simulink library "TOWER_MASTER"  (Simulink 8.8)
settings: Solver=ode45  StartTime=0.0  StopTime=10.0  RelTol=1e-3  EnableMultiTasking=on
undefined symbols (not defined in the file): AC, AC2THRESHOLD, BF_WD_MASTER, GAS_WD_MASTER, GASAC, SIXOSEM_F_WD_AC_MASTER
libraries: cdsEpicsOut x163, cdsFilt x111, cdsTP x68, cdsFiltCtrl x56, cdsEpicsIn x47, cdsMuxMatrix x14, cdsRms x14, TOWER_MASTER x11, STATE_BIO_MASTER x8, cdsEpicsBinIn x6, cdsFunctionCall x4, VIS_LIB x2
(part 1 of 19)
settings Model: SuppressorTable=22 serialization::archive 11 0 3 0 0 0 11 0  Creator=controls  LastModifiedBy=controls

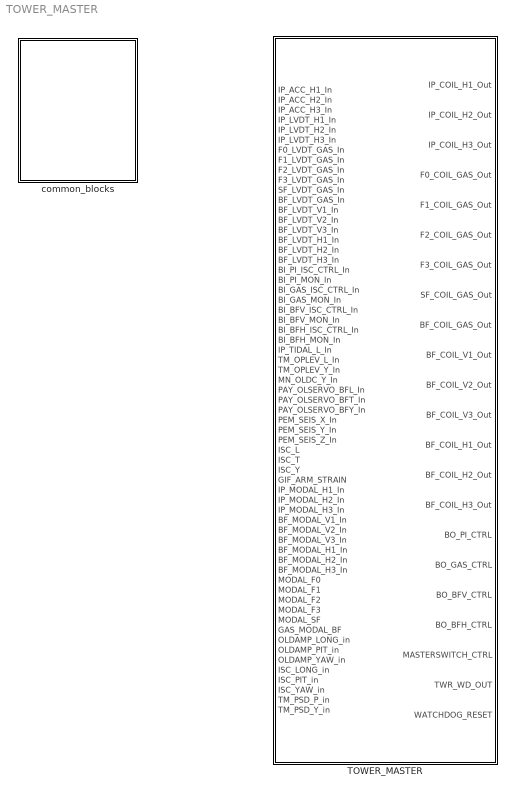
== system TOWER_MASTER ==
  TOWER_MASTER : Subsystem
  common_blocks : Subsystem

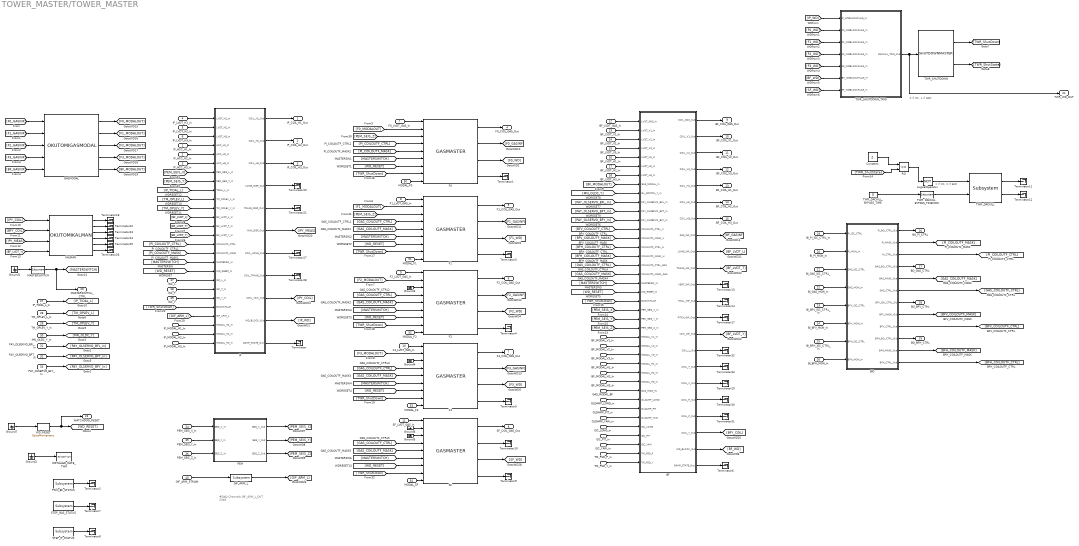
== system TOWER_MASTER/TOWER_MASTER ==
  note: 1 if OK, 0 if BAD
  note: 0 if OK, 1 if BAD
  note: #DAQ Channels
      | GIF_ARM_L_OUT 2048
  IP_ACC_H1_In : Inport
  IP_ACC_H2_In : Inport  Port=2
  IP_ACC_H3_In : Inport  Port=3
  IP_LVDT_H1_In : Inport  Port=4
  IP_LVDT_H2_In : Inport  Port=5
  IP_LVDT_H3_In : Inport  Port=6
  F0_LVDT_GAS_In : Inport  Port=7
  F1_LVDT_GAS_In : Inport  Port=8
  F2_LVDT_GAS_In : Inport  Port=9
  F3_LVDT_GAS_In : Inport  Port=10
  SF_LVDT_GAS_In : Inport  Port=11
  BF_LVDT_GAS_In : Inport  Port=12
  BF_LVDT_V1_In : Inport  Port=13
  BF_LVDT_V2_In : Inport  Port=14
  BF_LVDT_V3_In : Inport  Port=15
  BF_LVDT_H1_In : Inport  Port=16
  BF_LVDT_H2_In : Inport  Port=17
  BF_LVDT_H3_In : Inport  Port=18
  BI_PI_ISC_CTRL_In : Inport  Port=19
  BI_PI_MON_In : Inport  Port=20
  BI_GAS_ISC_CTRL_In : Inport  Port=21
  BI_GAS_MON_In : Inport  Port=22
  BI_BFV_ISC_CTRL_In : Inport  Port=23
  BI_BFV_MON_In : Inport  Port=24
  BI_BFH_ISC_CTRL_In : Inport  Port=25
  BI_BFH_MON_In : Inport  Port=26
  IP_TIDAL_L_In : Inport  Port=27
  TM_OPLEV_L_In : Inport  Port=28
  TM_OPLEV_Y_In : Inport  Port=29
  MN_OLDC_Y_In : Inport  Port=30
  PAY_OLSERVO_BFL_In : Inport  Port=31
  PAY_OLSERVO_BFT_In : Inport  Port=32
  PAY_OLSERVO_BFY_In : Inport  Port=33
  PEM_SEIS_X_In : Inport  Port=34
  PEM_SEIS_Y_In : Inport  Port=35
  PEM_SEIS_Z_In : Inport  Port=36
  ISC_L : Inport  Port=37
  ISC_T : Inport  Port=38
  ISC_Y : Inport  Port=39
  GIF_ARM_STRAIN : Inport  Port=40
  IP_MODAL_H1_In : Inport  Port=41
  IP_MODAL_H2_In : Inport  Port=42
  IP_MODAL_H3_In : Inport  Port=43
  BF_MODAL_V1_In : Inport  Port=44
  BF_MODAL_V2_In : Inport  Port=45
  BF_MODAL_V3_In : Inport  Port=46
  BF_MODAL_H1_In : Inport  Port=47
  BF_MODAL_H2_In : Inport  Port=48
  BF_MODAL_H3_In : Inport  Port=49
  MODAL_F0 : Inport  Port=50
  MODAL_F1 : Inport  Port=51
  MODAL_F2 : Inport  Port=52
  MODAL_F3 : Inport  Port=53
  MODAL_SF : Inport  Port=54
  GAS_MODAL_BF : Inport  Port=55
  OLDAMP_LONG_in : Inport  Port=56
  OLDAMP_PIT_in : Inport  Port=57
  OLDAMP_YAW_in : Inport  Port=58
  ISC_LONG_in : Inport  Port=59
  ISC_PIT_in : Inport  Port=60
  ISC_YAW_in : Inport  Port=61
  TM_PSD_P_in : Inport  Port=62
  TM_PSD_Y_in : Inport  Port=63
  BF : Subsystem
  BIO : Subsystem
  Constant : Constant  Value=2
  F{0..3} (4 alike) : TOWER_MASTER/common_blocks/GASMASTER
  GASMODAL : TOWER_MASTER/common_blocks/OKUTOMIGASMODAL
  GIF_ARM_L : cdsFilt/Subsystem  Tag=cdsFilt  Description=|
      | Purpose:                                                                                                                                                                                                                                  
      | Standard CDS IIR filter module.                                                                                                                                                                                                           
      |                                                                                                                                                                                                                                           
      | Operation:                                                                                                                                                                                                                                
      | Consists of 10 second order section IIR filters, plus a ramped gain stage. In FE code, also provides pre-defined test points and excitation channel inputs. The filter coefficients are defined in the LIGO system using the 'foton' tool.
      |                                                                                                                                                                                                                                           
      | Usage:                                                                                                                                                                                                                                    
      | Name the part with the desired filter module name.
      settings: AttributesFormatString=%<Tag>
  Ground{1..7} (7 alike) : Ground
  INSTALLED_DATE_TWR : cdsEpicsStringIn/EpicsStringIn  Tag=cdsEpicsStringIn  Description=cdsEpicsStringIn
      settings: AttributesFormatString=%<Tag>
  IP : Subsystem
  KALMAN : TOWER_MASTER/common_blocks/OKUTOMIKALMAN
  LogicalOperator : Logic  Operator=NOT  AllPortsSameDT=off  OutDataTypeStr=boolean
  MASTERSWITCH : cdsEpicsBinIn/Subsystem  Tag=cdsEpicsBinIn  Description=|
      | Purpose:                                                                            
      | Create an EPICS binary (0 or 1) input channel to the FE realtime controls.          
      |                                                                                     
      | Operation:                                                                          
      | Outputs value from an EPICS ai record. Value is binary input (bi Epics record type).
      |                                                                                     
      | Usage:                                                                              
      | Name the part with the desired EPICS channel name.
      settings: AttributesFormatString=%<Tag>
  PEM : Subsystem
  PICO_BF_STATUS : cdsEpicsIn/Subsystem  Tag=cdsEpicsIn  Description=|
      | Purpose:                                                                              
      | Create an EPICS input channel connection to the FE realtime controls.                 
      |                                                                                       
      | Operation:                                                                            
      | Outputs value from an EPICS ai record. Value is floating point with a precision of 3..
      |                                                                                       
      | Usage:                                                                                
      | Name the part with the desired EPICS channel name.
      settings: AttributesFormatString=%<Tag>
  RO : RelationalOperator  Operator===  OutDataTypeStr=boolean  RndMeth=Nearest
  SF : TOWER_MASTER/common_blocks/GASMASTER
  STEP_GAS_STATUS : cdsEpicsIn/Subsystem  Tag=cdsEpicsIn  Description=|
      | Purpose:                                                                              
      | Create an EPICS input channel connection to the FE realtime controls.                 
      |                                                                                       
      | Operation:                                                                            
      | Outputs value from an EPICS ai record. Value is floating point with a precision of 3..
      |                                                                                       
      | Usage:                                                                                
      | Name the part with the desired EPICS channel name.
      settings: AttributesFormatString=%<Tag>
  STEP_IP_STATUS : cdsEpicsIn/Subsystem  Tag=cdsEpicsIn  Description=|
      | Purpose:                                                                              
      | Create an EPICS input channel connection to the FE realtime controls.                 
      |                                                                                       
      | Operation:                                                                            
      | Outputs value from an EPICS ai record. Value is floating point with a precision of 3..
      |                                                                                       
      | Usage:                                                                                
      | Name the part with the desired EPICS channel name.
      settings: AttributesFormatString=%<Tag>
  TWR_DACKILL : cdsDacKill/Subsystem  Description=cdsDacKill
      settings: AttributesFormatString=%<Description>
  TWR_DACKILL_BYPASS_TIME : Constant  Value=0
  TWR_DACKILL_BYPASS_TIMEMON : cdsEpicsOut/Subsystem  Tag=cdsEpicsOutput  Description=|
      | Purpose:                                          
      | Output a FE signal to an EPICS channel.           
      |                                                   
      | Operation:                                        
      | Takes input value and passes it to EPICS record.  
      |                                                   
      | Usage:                                            
      | Name the part with the desired EPICS rrecord name.
      settings: AttributesFormatString=%<Tag>
  TWR_SHUTDOWN : TOWER_MASTER/common_blocks/SHUTDOWNMASTER
  TWR_SHUTDOWN_TRIG : Subsystem
  Terminator{,1..14,17..18,20..33} (31 alike) : Terminator
  WD_RESET : cdsEpicsMomentary/EpicsMomentary  Tag=cdsEpicsMomentary
      settings: AttributesFormatString=%<Tag>
  IP_COIL_H1_Out : Outport
  IP_COIL_H2_Out : Outport  Port=2
  IP_COIL_H3_Out : Outport  Port=3
  F0_COIL_GAS_Out : Outport  Port=4
  F1_COIL_GAS_Out : Outport  Port=5
  F2_COIL_GAS_Out : Outport  Port=6
  F3_COIL_GAS_Out : Outport  Port=7
  SF_COIL_GAS_Out : Outport  Port=8
  BF_COIL_GAS_Out : Outport  Port=9
  BF_COIL_V1_Out : Outport  Port=10
  BF_COIL_V2_Out : Outport  Port=11
  BF_COIL_V3_Out : Outport  Port=12
  BF_COIL_H1_Out : Outport  Port=13
  BF_COIL_H2_Out : Outport  Port=14
  BF_COIL_H3_Out : Outport  Port=15
  BO_PI_CTRL : Outport  Port=16
  BO_GAS_CTRL : Outport  Port=17
  BO_BFV_CTRL : Outport  Port=18
  BO_BFH_CTRL : Outport  Port=19
  MASTERSWITCH_CTRL : Outport  Port=20
  TWR_WD_OUT : Outport  Port=21
  WATCHDOG_RESET : Outport  Port=22
  wires:
  ISC_Y/1 -> IP/21(ISC_Y_in)
  ISC_T/1 -> IP/20(ISC_T_in)
  ISC_L/1 -> IP/19(ISC_L_in)
  GAS_MODAL_BF/1 -> BF/31(GAS_MOD_IN)
  BF_MODAL_H3_In/1 -> BF/30(MODAL_H3_In)
  BF_MODAL_H2_In/1 -> BF/29(MODAL_H2_In)
  BF_MODAL_H1_In/1 -> BF/28(MODAL_H1_In)
  BF_MODAL_V3_In/1 -> BF/27(MODAL_V3_In)
  BF_MODAL_V2_In/1 -> BF/26(MODAL_V2_In)
  BF_MODAL_V1_In/1 -> BF/25(MODAL_V1_In)
  [PEM_SEIS_Z] -> BF/24(PEM_SEIS_Z_In)
  [PEM_SEIS_Y] -> BF/23(PEM_SEIS_Y_In)
  [PEM_SEIS_X] -> BF/22(PEM_SEIS_X_In)
  [TWR_ShutDown] -> BF/21(BLOCKFLAG)
  [WD_RESET] -> BF/20(WD_RESET_In)
  [MASTERSWITCH] -> BF/19(MASTERSW_In)
  [GAS_COILOUTF_MASK] -> BF/18(COILOUTF_MASK_GAS)
  [GAS_COILOUTF_CTRL] -> BF/17(COILOUTF_CTRL_GAS)
  [BFH_COILOUTF_MASK] -> BF/16(COILOUTF_MASK_H)
  [BFH_COILOUTF_CTRL] -> BF/15(COILOUTF_CTRL_H)
  [BFV_COILOUTF_MASK] -> BF/14(COILOUTF_MASK_V)
  [BFV_COILOUTF_CTRL] -> BF/13(COILOUTF_CTRL_V)
  [PAY_OLSERVO_BFY_In] -> BF/12(PAY_OLSERVO_BFY_In)
  [PAY_OLSERVO_BFT_In] -> BF/11(PAY_OLSERVO_BFT_In)
  [PAY_OLSERVO_BFL_In] -> BF/10(PAY_OLSERVO_BFL_In)
  [MN_OLDC_Y] -> BF/9(OL_DCCTRL_Y_In)
  [BF_MODALOUT] -> BF/8(GAS_MODAL_In)
  BF_LVDT_H3_In/1 -> BF/7(LVDT_H3_In)
  BF_LVDT_H2_In/1 -> BF/6(LVDT_H2_In)
  BF_LVDT_H1_In/1 -> BF/5(LVDT_H1_In)
  BF_LVDT_V3_In/1 -> BF/4(LVDT_V3_In)
  BF_LVDT_V2_In/1 -> BF/3(LVDT_V2_In)
  BF_LVDT_V1_In/1 -> BF/2(LVDT_V1_In)
  BF_LVDT_GAS_In/1 -> BF/1(LVDT_GAS_In)
  TM_PSD_Y_in/1 -> BF/39(TM_PSD_Y)
  TM_PSD_P_in/1 -> BF/38(TM_PSD_P)
  ISC_PIT_in/1 -> BF/36(ISC_PIT)
  OLDAMP_YAW_in/1 -> BF/34(OLDAMP_YAW)
  OLDAMP_PIT_in/1 -> BF/33(OLDAMP_PIT)
  OLDAMP_LONG_in/1 -> BF/32(OLDAMP_LONG)
  ISC_YAW_in/1 -> BF/37(ISC_YAW)
  ISC_LONG_in/1 -> BF/35(ISC_LONG)
  [TWR_ShutDown] -> IP/22(BLOCKFLAG)
  [GIF_ARM_L] -> IP/23(GIF_ARM_L)
  MODAL_F3/1 -> F3/9
  MODAL_F2/1 -> F2/9
  MODAL_F1/1 -> F1/9
  MODAL_F0/1 -> F0/9
  IP_MODAL_H1_In/1 -> IP/24(MODAL_H1_In)
  IP_MODAL_H2_In/1 -> IP/25(MODAL_H2_In)
  IP_MODAL_H3_In/1 -> IP/26(MODAL_H3_In)
  RO/1 -> LogicalOperator/1
  [TWR_ShutState] -> RO/2
  Constant/1 -> RO/1
  TWR_SHUTDOWN/2 -> [TWR_ShutState]
  TWR_SHUTDOWN/1 -> [TWR_ShutDown]
  TWR_SHUTDOWN_TRIG/1(DACKILL_TRIG_Out) -> TWR_SHUTDOWN/1, TWR_WD_OUT/1
  TWR_DACKILL/2 -> Terminator12/1
  TWR_DACKILL/1 -> Terminator11/1
  TWR_DACKILL_BYPASS_TIME/1 -> TWR_DACKILL_BYPASS_TIMEMON/1
  TWR_DACKILL_BYPASS_TIMEMON/1 -> TWR_DACKILL/2
  LogicalOperator/1 -> TWR_DACKILL/1
  WD_RESET/1 -> [WD_RESET], WATCHDOG_RESET/1
  Ground7/1 -> WD_RESET/1
  MN_OLDC_Y_In/1 -> [MN_OLDC_Y]
  [IPY_MEAS] -> KALMAN/3
  [BF_LVDT_Y] -> KALMAN/4
  BF/20(COIL_Y_Out) -> [BFY_COIL]
  BF/17(COIL_V_Out) -> Terminator29/1
  BF/19(COIL_P_Out) -> Terminator31/1
  BF/18(COIL_R_Out) -> Terminator30/1
  BF/16(COIL_T_Out) -> Terminator33/1
  BF/15(COIL_L_Out) -> Terminator32/1
  BF/21(WD_BLOCK_Out) -> [BF_WD]
  BF/14(YAW_INF_Out) -> [BF_LVDT_Y]
  IP/11(DAMP_STATE_Out) -> Terminator/1
  IP/10(WD_BLOCK_Out) -> [IP_WD]
  IP/5(TRANS_DISP_Out) -> Terminator21/1
  IP/4(LONG_DISP_Out) -> Terminator20/1
  IP/9(COIL_YAW_Out) -> [IPY_COIL]
  IP/8(COIL_TRANS_Out) -> Terminator28/1
  IP/7(COIL_LONG_Out) -> Terminator27/1
  IP/6(YAW_DISP_Out) -> [IPY_MEAS]
  IP/3(COIL_H3_Out) -> IP_COIL_H3_Out/1
  KALMAN/6 -> Terminator26/1
  KALMAN/5 -> Terminator25/1
  KALMAN/4 -> Terminator24/1
  KALMAN/3 -> Terminator23/1
  KALMAN/2 -> Terminator22/1
  KALMAN/1 -> Terminator18/1
  [BFY_COIL] -> KALMAN/2
  [IPY_COIL] -> KALMAN/1
  BF/13(PITCH_INF_Out) -> Terminator17/1
  BF/12(ROLL_INF_Out) -> Terminator14/1
  BF/11(VERT_INF_Out) -> Terminator13/1
  BF/10(TRANS_INF_Out) -> [BF_LVDT_T]
  BF/9(LONG_INF_Out) -> [BF_LVDT_L]
  BF/8(GAS_INF_Out) -> [BF_GASINF]
  BF/7(COIL_H3_Out) -> BF_COIL_H3_Out/1
  BF/6(COIL_H2_Out) -> BF_COIL_H2_Out/1
  BF/5(COIL_H1_Out) -> BF_COIL_H1_Out/1
  BF/4(COIL_V3_Out) -> BF_COIL_V3_Out/1
  BF/3(COIL_V2_Out) -> BF_COIL_V2_Out/1
  BF/2(COIL_V1_Out) -> BF_COIL_V1_Out/1
  BF/1(COIL_GAS_Out) -> BF_COIL_GAS_Out/1
  [F3_MODALOUT] -> F3/2
  [F2_MODALOUT] -> F2/2
  [F1_MODALOUT] -> F1/2
  [F0_MODALOUT] -> F0/2
  GASMODAL/4 -> [F3_MODALOUT]
  GASMODAL/2 -> [F1_MODALOUT]
  GASMODAL/3 -> [F2_MODALOUT]
  GASMODAL/5 -> [BF_MODALOUT]
  GASMODAL/1 -> [F0_MODALOUT]
  [BF_GASINF] -> GASMODAL/5
  [F0_GASINF] -> GASMODAL/1
  [F1_GASINF] -> GASMODAL/2
  [F3_GASINF] -> GASMODAL/4
  [F2_GASINF] -> GASMODAL/3
  F3/2 -> [F3_GASINF]
  F2/2 -> [F2_GASINF]
  F1/2 -> [F1_GASINF]
  F0/2 -> [F0_GASINF]
  F3_LVDT_GAS_In/1 -> F3/1
  F2_LVDT_GAS_In/1 -> F2/1
  F1_LVDT_GAS_In/1 -> F1/1
  F0_LVDT_GAS_In/1 -> F0/1
  F0/3 -> [F0_WD]
  F0/4 -> Terminator1/1
  F0/1 -> F0_COIL_GAS_Out/1
  BI_BFH_MON_In/1 -> BIO/8(BFH_MON_In)
  BI_BFH_ISC_CTRL_In/1 -> BIO/7(BFH_ISC_CTRL)
  BIO/10(BFH_BO_CTRL_Out) -> BO_BFH_CTRL/1
  BIO/12(BFH_CTRL_Out) -> [BFH_COILOUTF_CTRL]
  BIO/11(BFH_MASK_Out) -> [BFH_COILOUTF_MASK]
  BIO/9(BFV_CTRL_Out) -> [BFV_COILOUTF_CTRL]
  BIO/6(GAS_CTRL_Out) -> [GAS_COILOUTF_CTRL]
  BIO/3(PI_CTRL_Out) -> [PI_COILOUTF_CTRL]
  BIO/8(BFV_MASK_Out) -> [BFV_COILOUTF_MASK]
  BIO/5(GAS_MASK_Out) -> [GAS_COILOUTF_MASK]
  BIO/2(PI_MASK_Out) -> [PI_COILOUTF_MASK]
  BIO/7(BFV_BO_CTRL_Out) -> BO_BFV_CTRL/1
  BIO/4(GAS_BO_CTRL_Out) -> BO_GAS_CTRL/1
  BIO/1(PI_BO_CTRL_Out) -> BO_PI_CTRL/1
  BI_PI_MON_In/1 -> BIO/2(PI_MON_In)
  BI_PI_ISC_CTRL_In/1 -> BIO/1(PI_ISC_CTRL)
  BI_GAS_MON_In/1 -> BIO/4(GAS_MON_In)
  BI_BFV_MON_In/1 -> BIO/6(BFV_MON_In)
  BI_GAS_ISC_CTRL_In/1 -> BIO/3(GAS_ISC_CTRL)
  BI_BFV_ISC_CTRL_In/1 -> BIO/5(BFV_ISC_CTRL)
  [BF_WD] -> TWR_SHUTDOWN_TRIG/6(BF_WDBLOCKFLAG_In)
  [F3_WD] -> TWR_SHUTDOWN_TRIG/5(F3_WDBLOCKFLAG_In)
  [F2_WD] -> TWR_SHUTDOWN_TRIG/4(F2_WDBLOCKFLAG_In)
  [F1_WD] -> TWR_SHUTDOWN_TRIG/3(F1_WDBLOCKFLAG_In)
  [F0_WD] -> TWR_SHUTDOWN_TRIG/2(F0_WDBLOCKFLAG_In)
  [IP_WD] -> TWR_SHUTDOWN_TRIG/1(IP_WDBLOCKFLAG_In)
  F3/4 -> Terminator5/1
  F2/4 -> Terminator4/1
  F1/4 -> Terminator3/1
  F3/1 -> F3_COIL_GAS_Out/1
  F2/1 -> F2_COIL_GAS_Out/1
  F1/1 -> F1_COIL_GAS_Out/1
  F3/3 -> [F3_WD]
  F2/3 -> [F2_WD]
  F1/3 -> [F1_WD]
  MASTERSWITCH/1 -> MASTERSWITCH_CTRL/1, [MASTERSWITCH]
  IP/2(COIL_H2_Out) -> IP_COIL_H2_Out/1
  IP/1(COIL_H1_Out) -> IP_COIL_H1_Out/1
  IP_ACC_H3_In/1 -> IP/6(ACC_H3_In)
  IP_LVDT_H3_In/1 -> IP/3(LVDT_H3_In)
  IP_ACC_H1_In/1 -> IP/4(ACC_H1_In)
  IP_LVDT_H1_In/1 -> IP/1(LVDT_H1_In)
  IP_ACC_H2_In/1 -> IP/5(ACC_H2_In)
  IP_LVDT_H2_In/1 -> IP/2(LVDT_H2_In)
  PAY_OLSERVO_BFY_In/1 -> [PAY_OLSERVO_BFY_In]
  BF/22(DAMP_STATE_Out) -> Terminator6/1
  PEM/1(SEIS_X_Out) -> [PEM_SEIS_X]
  [PEM_SEIS_X] -> IP/7(PEM_SEIS_L_In)
  PEM/2(SEIS_Y_Out) -> [PEM_SEIS_Y]
  PEM/3(SEIS_Z_Out) -> [PEM_SEIS_Z]
  [PEM_SEIS_Y] -> IP/8(PEM_SEIS_T_In)
  PAY_OLSERVO_BFL_In/1 -> [PAY_OLSERVO_BFL_In]
  PAY_OLSERVO_BFT_In/1 -> [PAY_OLSERVO_BFT_In]
  PEM_SEIS_Y_In/1 -> PEM/2(SEIS_Y_In)
  PEM_SEIS_X_In/1 -> PEM/1(SEIS_X_In)
  PEM_SEIS_Z_In/1 -> PEM/3(SEIS_Z_In)
  TM_OPLEV_L_In/1 -> [TM_OPLEV_L]
  TM_OPLEV_Y_In/1 -> [TM_OPLEV_Y]
  GIF_ARM_L/1 -> [GIF_ARM_L]
  GIF_ARM_STRAIN/1 -> GIF_ARM_L/1
  [MASTERSWITCH] -> F0/6
  [PI_COILOUTF_CTRL] -> F0/4
  [PI_COILOUTF_MASK] -> F0/5
  [WD_RESET] -> F0/7
  [TWR_ShutDown] -> F0/8
  [GAS_COILOUTF_CTRL] -> F1/4
  [GAS_COILOUTF_MASK] -> F1/5
  [MASTERSWITCH] -> F1/6
  [WD_RESET] -> F1/7
  [TWR_ShutDown] -> F1/8
  Ground3/1 -> F2/3
  [GAS_COILOUTF_MASK] -> F2/5
  [MASTERSWITCH] -> F2/6
  [WD_RESET] -> F2/7
  [GAS_COILOUTF_CTRL] -> F2/4
  [TWR_ShutDown] -> F2/8
  Ground4/1 -> F3/3
  [GAS_COILOUTF_CTRL] -> F3/4
  [GAS_COILOUTF_MASK] -> F3/5
  [MASTERSWITCH] -> F3/6
  [WD_RESET] -> F3/7
  [TWR_ShutDown] -> F3/8
  [PEM_SEIS_Z] -> F1/3
  [PEM_SEIS_Z] -> F0/3
  Ground1/1 -> MASTERSWITCH/1
  [IP_TIDAL_L] -> IP/9(TIDAL_L_In)
  [BF_LVDT_Y] -> IP/14(BF_LVDT_Y_In)
  [BF_LVDT_T] -> IP/13(BF_LVDT_T_In)
  [BF_LVDT_L] -> IP/12(BF_LVDT_L_In)
  [TM_OPLEV_L] -> IP/10(TM_OPLEV_L_In)
  [TM_OPLEV_Y] -> IP/11(TM_OPLEV_Y_In)
  [MASTERSWITCH] -> IP/17(MASTERSW_In)
  [PI_COILOUTF_CTRL] -> IP/15(COILOUTF_CTRL)
  [PI_COILOUTF_MASK] -> IP/16(COILOUTF_MASK)
  [WD_RESET] -> IP/18(WD_RESET_In)
  IP_TIDAL_L_In/1 -> [IP_TIDAL_L]
  PICO_BF_STATUS/1 -> Terminator2/1
  STEP_GAS_STATUS/1 -> Terminator7/1
  STEP_IP_STATUS/1 -> Terminator8/1
  Ground2/1 -> INSTALLED_DATE_TWR/1
  MODAL_SF/1 -> SF/9
  Ground6/1 -> SF/2
  SF/2 -> Terminator10/1
  SF_LVDT_GAS_In/1 -> SF/1
  SF/4 -> Terminator9/1
  SF/1 -> SF_COIL_GAS_Out/1
  SF/3 -> [SF_WD]
  Ground5/1 -> SF/3
  [GAS_COILOUTF_CTRL] -> SF/4
  [GAS_COILOUTF_MASK] -> SF/5
  [MASTERSWITCH] -> SF/6
  [WD_RESET] -> SF/7
  [TWR_ShutDown] -> SF/8
  [SF_WD] -> TWR_SHUTDOWN_TRIG/7(SF_WDBLOCKFLAG_In)

== system TOWER_MASTER/common_blocks ==
  note: TWR
      | Common
  note: In-preparation
  note: Only One
  note: Stage
      | Common
  note: VIS
      | Common
  BIO : Subsystem
  BIODECODE : Subsystem
  BIOENCODE : Subsystem
  GASMASTER : Subsystem
  OKUTOMIGASMODAL : Subsystem
  OKUTOMIKALMAN : Subsystem
  SHUTDOWNMASTER : Subsystem
  WDMONMASTER : Subsystem

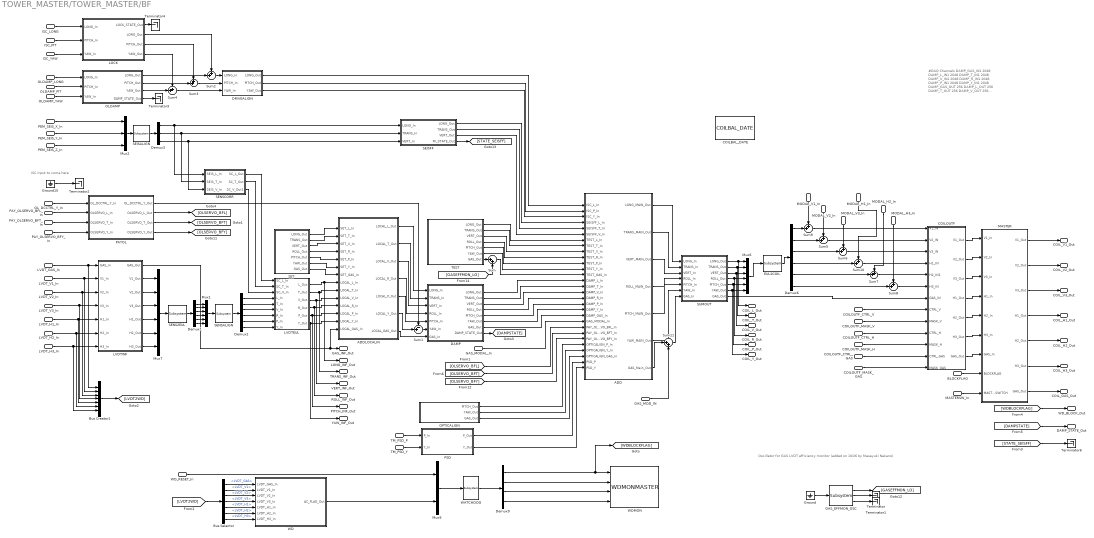
== system TOWER_MASTER/TOWER_MASTER/BF ==
  note: Oscillator for GAS LVDT efficiency monitor (added on 10/26 by Masayuki Nakano)
  note: ISC input to come here
  note: #DAQ Channels
      | DAMP_GAS_IN1 2048
      | DAMP_L_IN1 2048
      | DAMP_T_IN1 2048
      | DAMP_V_IN1 2048
      | DAMP_R_IN1 2048
      | DAMP_P_IN1 2048
      | DAMP_Y_IN1 2048
      | DAMP_GAS_OUT 256
      | DAMP_L_OUT 256
      | DAMP_T_OUT 256
      | DAMP_V_OUT 256
      | DAMP_R_OUT 256
      | DAMP_P_OUT 256
      | DAMP_Y_OUT 256
      | LVDTINF_GAS_IN1 2048
  LVDT_GAS_In : Inport
  LVDT_V1_In : Inport  Port=2
  LVDT_V2_In : Inport  Port=3
  LVDT_V3_In : Inport  Port=4
  LVDT_H1_In : Inport  Port=5
  LVDT_H2_In : Inport  Port=6
  LVDT_H3_In : Inport  Port=7
  GAS_MODAL_In : Inport  Port=8
  OL_DCCTRL_Y_In : Inport  Port=9
  PAY_OLSERVO_BFL_In : Inport  Port=10
  PAY_OLSERVO_BFT_In : Inport  Port=11
  PAY_OLSERVO_BFY_In : Inport  Port=12
  COILOUTF_CTRL_V : Inport  Port=13
  COILOUTF_MASK_V : Inport  Port=14
  COILOUTF_CTRL_H : Inport  Port=15
  COILOUTF_MASK_H : Inport  Port=16
  COILOUTF_CTRL_GAS : Inport  Port=17
  COILOUTF_MASK_GAS : Inport  Port=18
  MASTERSW_In : Inport  Port=19
  WD_RESET_In : Inport  Port=20
  BLOCKFLAG : Inport  Port=21
  PEM_SEIS_X_In : Inport  Port=22
  PEM_SEIS_Y_In : Inport  Port=23
  PEM_SEIS_Z_In : Inport  Port=24
  MODAL_V1_In : Inport  Port=25
  MODAL_V2_In : Inport  Port=26
  MODAL_V3_In : Inport  Port=27
  MODAL_H1_In : Inport  Port=28
  MODAL_H2_In : Inport  Port=29
  MODAL_H3_In : Inport  Port=30
  GAS_MOD_IN : Inport  Port=31
  OLDAMP_LONG : Inport  Port=32
  OLDAMP_PIT : Inport  Port=33
  OLDAMP_YAW : Inport  Port=34
  ISC_LONG : Inport  Port=35
  ISC_PIT : Inport  Port=36
  ISC_YAW : Inport  Port=37
  TM_PSD_P : Inport  Port=38
  TM_PSD_Y : Inport  Port=39
  ADD : Subsystem
  ADDLOCALIN : Subsystem
  Bus Creator1 : BusCreator  Inputs='LVDT_GAS','LVDT_V1','LVDT_V2','LVDT_V3','LVDT_H1','LVDT_H2','LVDT_H3'
  Bus Selector : BusSelector  OutputSignals=LVDT_GAS,LVDT_V1,LVDT_V2,LVDT_V3,LVDT_H1,LVDT_H2,LVDT_H3
  COILBAL_DATE : VIS_LIB/COILBAL_DATE
  COILOUTF : Subsystem
  DAMP : Subsystem
  DRIVEALIGN : Subsystem
  Demux1 : Demux  Outputs=6
  Demux2 : Demux  Outputs=6
  Demux3 : Demux  Outputs=3
  Demux6 : Demux  Outputs=6
  Demux9 : Demux
  EUL2COIL : cdsMuxMatrix/Subsystem  Tag=cdsMuxMatrix  Description=|
      | ADL=SUS_INMATRIX.adl
      | SCRIPT=generate_KisselButton.py 4 5 #CHANNEL# > #TARGET_DIR#/#FULL_PART_NAME#_KB.adl
      settings: AttributesFormatString=%<Tag>
  GAS_EFFMON_OSC : cdsOsc/Subsystem  Tag=cdsOsc  Description=Oscillator
      settings: AttributesFormatString=%<Tag>
  Ground : Ground
  Ground15 : Ground
  LOCK : Subsystem
  LVDTEUL : Subsystem
  LVDTINF : Subsystem
  MASTER : Subsystem
  Mux1 : Mux  Inputs=6
  Mux2 : Mux  Inputs=3
  Mux6 : Mux  Inputs=6
  Mux7 : Mux  Inputs=6
  Mux9 : Mux  Inputs=2
  OLDAMP : Subsystem
  OPTICALIGN : Subsystem
  PAYOL : Subsystem
  PSD : Subsystem
  SEISALIGN : cdsMuxMatrix/Subsystem  Tag=cdsMuxMatrix  Description=|
      | ADL=SUS_INMATRIX.adl
      | SCRIPT=generate_KisselButton.py 4 5 #CHANNEL# > #TARGET_DIR#/#FULL_PART_NAME#_KB.adl
      settings: AttributesFormatString=%<Tag>
  SEISFF : Subsystem
  SENS2EUL : cdsMuxMatrix/Subsystem  Tag=cdsMuxMatrix  Description=Any size matrix. Inputs and outputs must be connected using Mux and Demux parts.
      settings: AttributesFormatString=%<Tag>
  SENSALIGN : cdsMuxMatrix/Subsystem  Tag=cdsMuxMatrix  Description=Any size matrix. Inputs and outputs must be connected using Mux and Demux parts.
      settings: AttributesFormatString=%<Tag>
  SENSCORR : Subsystem
  SET : Subsystem
  SUMOUT : Subsystem
  Sum : Sum  Inputs=|++
  Sum1 : Sum  Inputs=-+|
  Sum{2..10} (9 alike) : Sum  Inputs=++|
  Sum11 : Sum  Inputs=|++
  TEST : Subsystem
  Terminator{,1..4,6} (6 alike) : Terminator
  WATCHDOG : cdsFunctionCall/Subsystem  Tag=cdsFunctionCall  Description=inline OSEMWATCHDOG /opt/rtcds/userapps/release/vis/common/src/WATCHDOG.c
      settings: AttributesFormatString=%<Tag>\n%<Description>
  WD : Subsystem
  WDMON : TOWER_MASTER/common_blocks/WDMONMASTER
  COIL_GAS_Out : Outport
  COIL_V1_Out : Outport  Port=2
  COIL_V2_Out : Outport  Port=3
  COIL_V3_Out : Outport  Port=4
  COIL_H1_Out : Outport  Port=5
  COIL_H2_Out : Outport  Port=6
  COIL_H3_Out : Outport  Port=7
  GAS_INF_Out : Outport  Port=8
  LONG_INF_Out : Outport  Port=9
  TRANS_INF_Out : Outport  Port=10
  VERT_INF_Out : Outport  Port=11
  ROLL_INF_Out : Outport  Port=12
  PITCH_INF_Out : Outport  Port=13
  YAW_INF_Out : Outport  Port=14
  COIL_L_Out : Outport  Port=15
  COIL_T_Out : Outport  Port=16
  COIL_V_Out : Outport  Port=17
  COIL_R_Out : Outport  Port=18
  COIL_P_Out : Outport  Port=19
  COIL_Y_Out : Outport  Port=20
  WD_BLOCK_Out : Outport  Port=21
  DAMP_STATE_Out : Outport  Port=22
  wires:
  ADD/1(LONG_MAIN_Out) -> SUMOUT/1(LONG_In)
  ADD/6(YAW_MAIN_Out) -> SUMOUT/6(YAW_In)
  ADD/2(TRANS_MAIN_Out) -> SUMOUT/2(TRANS_In)
  ADD/5(PITCH_MAIN_Out) -> SUMOUT/5(PITCH_In)
  ADD/3(VERT_MAIN_Out) -> SUMOUT/3(VERT_In)
  ADD/4(ROLL_MAIN_Out) -> SUMOUT/4(ROLL_In)
  SUMOUT/7(GAS_Out) -> COILOUTF/7(GAS_IN)
  SUMOUT/5(PITCH_Out) -> Mux6/5, COIL_P_Out/1
  SUMOUT/4(ROLL_Out) -> Mux6/4, COIL_R_Out/1
  SUMOUT/2(TRANS_Out) -> Mux6/2, COIL_T_Out/1
  SUMOUT/3(VERT_Out) -> Mux6/3, COIL_V_Out/1
  SUMOUT/6(YAW_Out) -> Mux6/6, COIL_Y_Out/1
  SUMOUT/1(LONG_Out) -> Mux6/1, COIL_L_Out/1
  PAYOL/2(OLSERVO_L_Out) -> [OLSERVO_BFL]
  PAYOL/3(OLSERVO_T_Out) -> [OLSERVO_BFT]
  PAY_OLSERVO_BFT_In/1 -> PAYOL/3(OLSERVO_T_In)
  PAY_OLSERVO_BFL_In/1 -> PAYOL/2(OLSERVO_L_In)
  [OLSERVO_BFT] -> ADD/23(PAY_OLSERVO_BFT_In)
  [OLSERVO_BFL] -> ADD/22(PAY_OLSERVO_BFL_In)
  Sum1/1 -> DAMP/6(YAW_In)
  LVDTINF/1(GAS_Out) -> ADDLOCALIN/14(LOCAL_GAS_In), GAS_INF_Out/1
  ADDLOCALIN/6(LOCAL_Y_Out) -> Sum1/2
  ADDLOCALIN/7(LOCAL_GAS_Out) -> DAMP/7(GAS_In)
  SET/6(YAW_Out) -> ADDLOCALIN/6(SET_Y_In)
  SET/4(ROLL_Out) -> ADDLOCALIN/4(SET_R_In)
  SET/1(LONG_Out) -> ADDLOCALIN/1(SET_L_In)
  SET/5(PITCH_Out) -> ADDLOCALIN/5(SET_P_In)
  SET/7(GAS_Out) -> ADDLOCALIN/7(SET_GAS_In)
  SET/3(VERT_Out) -> ADDLOCALIN/3(SET_V_In)
  SET/2(TRANS_Out) -> ADDLOCALIN/2(SET_T_In)
  Demux2/6 -> LVDTEUL/9(Y_In)
  Demux2/5 -> LVDTEUL/8(P_In)
  Demux2/4 -> LVDTEUL/7(R_In)
  [STATE_SEISFF] -> Terminator6/1
  Sum/1 -> ADD/13(TEST_GAS_In)
  TEST/6(YAW_Out) -> ADD/12(TEST_Y_In)
  TEST/5(PITCH_Out) -> ADD/11(TEST_P_In)
  TEST/4(ROLL_Out) -> ADD/10(TEST_R_In)
  TEST/3(VERT_Out) -> ADD/9(TEST_V_In)
  TEST/2(TRANS_Out) -> ADD/8(TEST_T_In)
  TEST/1(LONG_Out) -> ADD/7(TEST_L_In)
  Demux3/3 -> SENSCORR/3(SEIS_V_In), SEISFF/3(VERT_In)
  PEM_SEIS_Z_In/1 -> Mux2/3
  Demux3/1 -> SENSCORR/1(SEIS_L_In), SEISFF/1(LONG_In)
  Demux3/2 -> SENSCORR/2(SEIS_T_In), SEISFF/2(TRANS_In)
  SEISALIGN/1 -> Demux3/1
  Mux2/1 -> SEISALIGN/1
  PEM_SEIS_X_In/1 -> Mux2/1
  PEM_SEIS_Y_In/1 -> Mux2/2
  SEISFF/4(FF_STATE_Out) -> [STATE_SEISFF]
  [OLSERVO_BFY] -> ADD/24(PAY_OLSERVO_BFY_In)
  PAYOL/4(OLSERVO_Y_Out) -> [OLSERVO_BFY]
  PAY_OLSERVO_BFY_In/1 -> PAYOL/4(OLSERVO_Y_In)
  OL_DCCTRL_Y_In/1 -> PAYOL/1(OL_DCCTRL_Y_In)
  GAS_MODAL_In/1 -> ADD/21(GAS_MODAL_In)
  Mux7/1 -> SENS2EUL/1
  Mux6/1 -> EUL2COIL/1
  EUL2COIL/1 -> Demux6/1
  MASTER/1(V1_Out) -> COIL_V1_Out/1
  MASTER/2(V2_Out) -> COIL_V2_Out/1
  MASTER/3(V3_Out) -> COIL_V3_Out/1
  WD_RESET_In/1 -> Mux9/1
  WD/1(AC_FLAG_Out) -> Mux9/2
  [LVDT2WD] -> Bus Selector/1
  Demux9/1 -> WDMON/1, [WDBLOCKFLAG]
  Demux9/2 -> WDMON/2
  Demux9/3 -> WDMON/3
  Demux9/4 -> WDMON/4
  Mux9/1 -> WATCHDOG/1
  WATCHDOG/1 -> Demux9/1
  LVDT_V1_In/1 -> Bus Creator1/2, LVDTINF/2(V1_In)
  LVDT_V2_In/1 -> Bus Creator1/3, LVDTINF/3(V2_In)
  LVDT_V3_In/1 -> Bus Creator1/4, LVDTINF/4(V3_In)
  LVDT_H1_In/1 -> LVDTINF/5(H1_In), Bus Creator1/5
  LVDT_H2_In/1 -> LVDTINF/6(H2_In), Bus Creator1/6
  LVDT_H3_In/1 -> LVDTINF/7(H3_In), Bus Creator1/7
  Bus Creator1/1 -> [LVDT2WD]
  COILOUTF_CTRL_V/1 -> COILOUTF/8(CTRL_V)
  COILOUTF_MASK_V/1 -> COILOUTF/9(MASK_V)
  LVDT_GAS_In/1 -> Bus Creator1/1, LVDTINF/1(GAS_In)
  MASTER/4(H1_Out) -> COIL_H1_Out/1
  Bus Selector/1 -> WD/1(LVDT_GAS_In)  "<LVDT_GAS>"
  SENS2EUL/1 -> Demux1/1
  Demux1/1 -> Mux1/1
  Demux1/2 -> Mux1/2
  Demux1/3 -> Mux1/3
  Demux1/4 -> Mux1/4
  Demux1/5 -> Mux1/5
  Demux1/6 -> Mux1/6
  Mux1/1 -> SENSALIGN/1
  SENSALIGN/1 -> Demux2/1
  LVDTINF/2(V1_Out) -> Mux7/1
  LVDTINF/3(V2_Out) -> Mux7/2
  LVDTINF/4(V3_Out) -> Mux7/3
  DAMP/8(DAMP_STATE_Out) -> [DAMPSTATE]
  DAMP/7(GAS_Out) -> ADD/20(DAMP_GAS_In)
  DAMP/6(YAW_Out) -> ADD/19(DAMP_Y_In)
  DAMP/5(PITCH_Out) -> ADD/18(DAMP_P_In)
  DAMP/4(ROLL_Out) -> ADD/17(DAMP_R_In)
  DAMP/3(VERT_Out) -> ADD/16(DAMP_V_In)
  DAMP/2(TRANS_Out) -> ADD/15(DAMP_T_In)
  DAMP/1(LONG_Out) -> ADD/14(DAMP_L_In)
  COILOUTF/5(H2_Out) -> MASTER/5(H2_In)
  COILOUTF/6(H3_Out) -> MASTER/6(H3_In)
  COILOUTF/7(GAS_Out) -> MASTER/7(GAS_In)
  COILOUTF/1(V1_Out) -> MASTER/1(V1_In)
  COILOUTF/2(V2_Out) -> MASTER/2(V2_In)
  COILOUTF/3(V3_Out) -> MASTER/3(V3_In)
  COILOUTF/4(H1_Out) -> MASTER/4(H1_In)
  BLOCKFLAG/1 -> MASTER/8(BLOCKFLAG)
  MASTERSW_In/1 -> MASTER/9(MASTERSWITCH)
  MASTER/5(H2_Out) -> COIL_H2_Out/1
  MASTER/6(H3_Out) -> COIL_H3_Out/1
  MASTER/7(GAS_Out) -> COIL_GAS_Out/1
  [WDBLOCKFLAG] -> WD_BLOCK_Out/1
  [DAMPSTATE] -> DAMP_STATE_Out/1
  Bus Selector/2 -> WD/2(LVDT_V1_In)  "<LVDT_V1>"
  Bus Selector/3 -> WD/3(LVDT_V2_In)  "<LVDT_V2>"
  Bus Selector/4 -> WD/4(LVDT_V3_In)  "<LVDT_V3>"
  Bus Selector/5 -> WD/5(LVDT_H1_In)  "<LVDT_H1>"
  Bus Selector/6 -> WD/6(LVDT_H2_In)  "<LVDT_H2>"
  Bus Selector/7 -> WD/7(LVDT_H3_In)  "<LVDT_H3>"
  LVDTINF/5(H1_Out) -> Mux7/4
  LVDTINF/6(H2_Out) -> Mux7/5
  LVDTINF/7(H3_Out) -> Mux7/6
  COILOUTF_CTRL_H/1 -> COILOUTF/10(CTRL_H)
  COILOUTF_MASK_H/1 -> COILOUTF/11(MASK_H)
  COILOUTF_CTRL_GAS/1 -> COILOUTF/12(CTRL_GAS)
  COILOUTF_MASK_GAS/1 -> COILOUTF/13(MASK_GAS)
  GAS_EFFMON_OSC/1 -> [GASEFFMON_LO]
  TEST/7(GAS_Out) -> Sum/1
  [GASEFFMON_LO] -> Sum/2
  Ground/1 -> GAS_EFFMON_OSC/1
  GAS_EFFMON_OSC/2 -> Terminator/1
  GAS_EFFMON_OSC/3 -> Terminator1/1
  Ground15/1 -> Terminator2/1
  Sum9/1 -> COILOUTF/1(V1_IN)
  MODAL_V1_In/1 -> Sum9/1
  Sum5/1 -> COILOUTF/2(V2_IN)
  MODAL_V2_In/1 -> Sum5/1
  Demux6/2 -> Sum5/2
  Sum6/1 -> COILOUTF/3(V3_IN)
  MODAL_V3_In/1 -> Sum6/1
  Demux6/3 -> Sum6/2
  Sum10/1 -> COILOUTF/4(H1_IN)
  MODAL_H1_In/1 -> Sum10/1
  Demux6/4 -> Sum10/2
  Sum7/1 -> COILOUTF/5(H2_IN1)
  MODAL_H2_In/1 -> Sum7/1
  Demux6/5 -> Sum7/2
  Sum8/1 -> COILOUTF/6(H3_IN)
  MODAL_H3_In/1 -> Sum8/1
  Demux6/6 -> Sum8/2
  Demux6/1 -> Sum9/2
  ADD/7(GAS_Main_Out) -> Sum11/1
  Sum11/1 -> SUMOUT/7(GAS_In)
  GAS_MOD_IN/1 -> Sum11/2
  Demux2/1 -> LVDTEUL/4(L_In)
  Demux2/3 -> LVDTEUL/6(V_In)
  SENSCORR/1(SC_L_Out) -> LVDTEUL/1(SC_L_In)
  SENSCORR/2(SC_T_Out) -> LVDTEUL/2(SC_T_In)
  SENSCORR/3(SC_V_Out1) -> LVDTEUL/3(SC_V_In)
  Demux2/2 -> LVDTEUL/5(T_In)
  ADDLOCALIN/5(LOCAL_P_Out) -> DAMP/5(PITCH_In)
  ADDLOCALIN/4(LOCAL_R_Out) -> DAMP/4(ROLL_In)
  ADDLOCALIN/3(LOCAL_V_Out) -> DAMP/3(VERT_In)
  ADDLOCALIN/2(LOCAL_T_Out) -> DAMP/2(TRANS_In)
  ADDLOCALIN/1(LOCAL_L_Out) -> DAMP/1(LONG_In)
  PAYOL/1(OL_DCCTRL_Y_Out) -> Sum1/1
  LVDTEUL/1(L_Out) -> LONG_INF_Out/1, ADDLOCALIN/8(LOCAL_L_In)
  LVDTEUL/2(T_Out) -> TRANS_INF_Out/1, ADDLOCALIN/9(LOCAL_T_In)
  LVDTEUL/3(V_Out) -> VERT_INF_Out/1, ADDLOCALIN/10(LOCAL_V_In)
  LVDTEUL/4(R_Out) -> ROLL_INF_Out/1, ADDLOCALIN/11(LOCAL_R_In)
  LVDTEUL/5(P_Out) -> PITCH_INF_Out/1, ADDLOCALIN/12(LOCAL_P_In)
  LVDTEUL/6(Y_Out) -> YAW_INF_Out/1, ADDLOCALIN/13(LOCAL_Y_In)
  OLDAMP/4(DAMP_STATE_Out) -> Terminator3/1
  OLDAMP_YAW/1 -> OLDAMP/3(YAW_In)
  OLDAMP_PIT/1 -> OLDAMP/2(PITCH_In)
  OLDAMP_LONG/1 -> OLDAMP/1(LONG_In)
  ISC_YAW/1 -> LOCK/3(YAW_In)
  ISC_PIT/1 -> LOCK/2(PITCH_In)
  ISC_LONG/1 -> LOCK/1(LONG_In)
  Sum2/1 -> DRIVEALIGN/1(LONG_In)
  OLDAMP/1(LONG_Out) -> Sum2/2
  LOCK/2(LONG_Out) -> Sum2/1
  OLDAMP/2(PITCH_Out) -> Sum3/2
  OLDAMP/3(YAW_Out) -> Sum4/2
  Sum4/1 -> DRIVEALIGN/3(YAW_In)
  LOCK/3(PITCH_Out) -> Sum3/1
  LOCK/4(YAW_Out) -> Sum4/1
  Sum3/1 -> DRIVEALIGN/2(PITCH_In)
  LOCK/1(LOCK_STATE_Out) -> Terminator4/1
  SEISFF/3(VERT_Out) -> ADD/6(SEISFF_V_In)
  SEISFF/2(TRANS_Out) -> ADD/5(SEISFF_T_In)
  SEISFF/1(LONG_Out) -> ADD/4(SEISFF_L_In)
  DRIVEALIGN/3(YAW_Out) -> ADD/3(ISC_Y_In)
  DRIVEALIGN/2(PITCH_Out) -> ADD/2(ISC_P_In)
  DRIVEALIGN/1(LONG_Out) -> ADD/1(ISC_L_In)
  OPTICALIGN/1(PITCH_Out) -> ADD/25(OPTICALIGN_P_In)
  OPTICALIGN/2(YAW_Out) -> ADD/26(OPTICALIGN_Y_In)
  OPTICALIGN/3(GAS_Out) -> ADD/27(OPTICALIGN_GAS_In)
  PSD/1(P_Out) -> ADD/28(PSD_P)
  PSD/2(Y_Out) -> ADD/29(PSD_Y)
  TM_PSD_P/1 -> PSD/1(P_In)
  TM_PSD_Y/1 -> PSD/2(Y_In)

== system TOWER_MASTER/TOWER_MASTER/BIO ==
  note: 12 Bit Word
  note: 12 Bit Word
  note: 12 Bit Word
  note: 12 Bit Word
  note: 12 Bit Word
  note: 12 Bit Word
  note: 12 Bit Word
  note: 12 Bit Word
  PI_ISC_CTRL : Inport
  PI_MON_In : Inport  Port=2
  GAS_ISC_CTRL : Inport  Port=3
  GAS_MON_In : Inport  Port=4
  BFV_ISC_CTRL : Inport  Port=5
  BFV_MON_In : Inport  Port=6
  BFH_ISC_CTRL : Inport  Port=7
  BFH_MON_In : Inport  Port=8
  BFH : STATE_BIO_MASTER/UIM_BIO_MASTER
  BFV : STATE_BIO_MASTER/UIM_BIO_MASTER
  GAS : STATE_BIO_MASTER/UIM_BIO_MASTER
  PI : STATE_BIO_MASTER/UIM_BIO_MASTER
  PI_BO_CTRL_Out : Outport
  PI_MASK_Out : Outport  Port=2
  PI_CTRL_Out : Outport  Port=3
  GAS_BO_CTRL_Out : Outport  Port=4
  GAS_MASK_Out : Outport  Port=5
  GAS_CTRL_Out : Outport  Port=6
  BFV_BO_CTRL_Out : Outport  Port=7
  BFV_MASK_Out : Outport  Port=8
  BFV_CTRL_Out : Outport  Port=9
  BFH_BO_CTRL_Out : Outport  Port=10
  BFH_MASK_Out : Outport  Port=11
  BFH_CTRL_Out : Outport  Port=12
  wires:
  BFH/3 -> BFH_BO_CTRL_Out/1
  BFH/2 -> BFH_CTRL_Out/1
  BFH/1 -> BFH_MASK_Out/1
  BFH_MON_In/1 -> BFH/2
  BFH_ISC_CTRL/1 -> BFH/1
  BFV/3 -> BFV_BO_CTRL_Out/1
  BFV/2 -> BFV_CTRL_Out/1
  BFV/1 -> BFV_MASK_Out/1
  BFV_MON_In/1 -> BFV/2
  BFV_ISC_CTRL/1 -> BFV/1
  PI/2 -> PI_CTRL_Out/1
  PI/1 -> PI_MASK_Out/1
  PI/3 -> PI_BO_CTRL_Out/1
  PI_MON_In/1 -> PI/2
  PI_ISC_CTRL/1 -> PI/1
  GAS/2 -> GAS_CTRL_Out/1
  GAS/1 -> GAS_MASK_Out/1
  GAS/3 -> GAS_BO_CTRL_Out/1
  GAS_MON_In/1 -> GAS/2
  GAS_ISC_CTRL/1 -> GAS/1

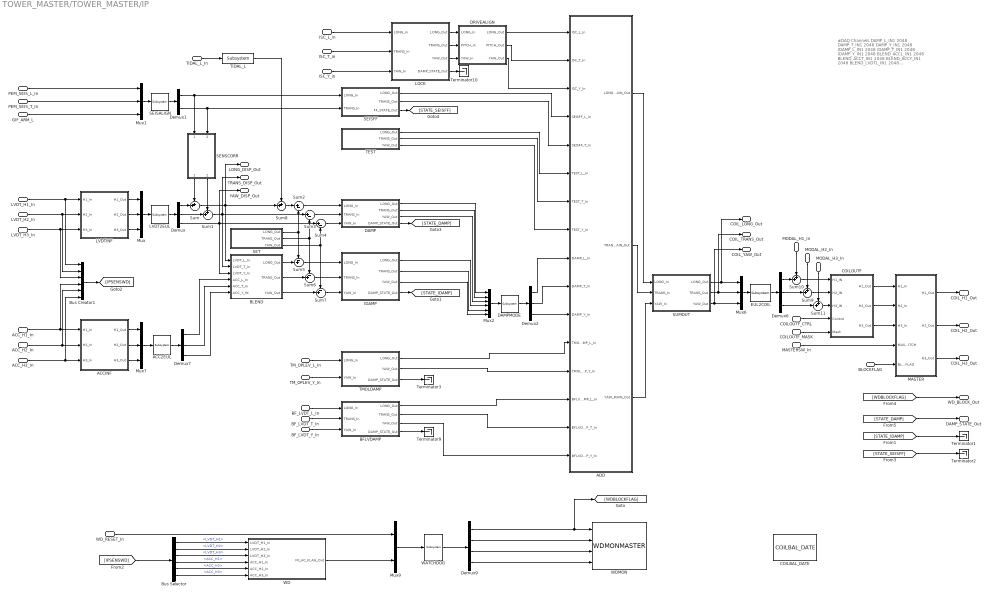
== system TOWER_MASTER/TOWER_MASTER/IP ==
  note: #DAQ Channels
      | DAMP_L_IN1 2048
      | DAMP_T_IN1 2048
      | DAMP_Y_IN1 2048
      | IDAMP_L_IN1 2048
      | IDAMP_T_IN1 2048
      | IDAMP_Y_IN1 2048
      | BLEND_ACCL_IN1 2048
      | BLEND_ACCT_IN1 2048
      | BLEND_ACCY_IN1 2048
      | BLEND_LVDTL_IN1 2048
      | BLEND_LVDTT_IN1 2048
      | BLEND_LVDTY_IN1 2048
      | DAMP_L_OUT 256
      | DAMP_T_OUT 256
      | DAMP_Y_OUT 256
      | IDAMP_L_OUT 256
      | IDAMP_T_OUT 256
      | IDAMP_Y_OUT 256
      | SEISFF_L_OUT 256
      | SEISFF_T_OUT 256
      | LOCK_L_OUT 256
      | TIDAL_L_OUT 32
  LVDT_H1_In : Inport
  LVDT_H2_In : Inport  Port=2
  LVDT_H3_In : Inport  Port=3
  ACC_H1_In : Inport  Port=4
  ACC_H2_In : Inport  Port=5
  ACC_H3_In : Inport  Port=6
  PEM_SEIS_L_In : Inport  Port=7
  PEM_SEIS_T_In : Inport  Port=8
  TIDAL_L_In : Inport  Port=9
  TM_OPLEV_L_In : Inport  Port=10
  TM_OPLEV_Y_In : Inport  Port=11
  BF_LVDT_L_In : Inport  Port=12
  BF_LVDT_T_In : Inport  Port=13
  BF_LVDT_Y_In : Inport  Port=14
  COILOUTF_CTRL : Inport  Port=15
  COILOUTF_MASK : Inport  Port=16
  MASTERSW_In : Inport  Port=17
  WD_RESET_In : Inport  Port=18
  ISC_L_in : Inport  Port=19
  ISC_T_in : Inport  Port=20
  ISC_Y_in : Inport  Port=21
  BLOCKFLAG : Inport  Port=22
  GIF_ARM_L : Inport  Port=23
  MODAL_H1_In : Inport  Port=24
  MODAL_H2_In : Inport  Port=25
  MODAL_H3_In : Inport  Port=26
  ACC2EUL : cdsMuxMatrix/Subsystem  Tag=cdsMuxMatrix  Description=|
      | ADL=SUS_INMATRIX.adl
      | SCRIPT=generate_KisselButton.py 4 5 #CHANNEL# > #TARGET_DIR#/#FULL_PART_NAME#_KB.adl
      settings: AttributesFormatString=%<Tag>
  ACCINF : Subsystem
  ADD : Subsystem
  BFLVDAMP : Subsystem
  BLEND : Subsystem
  Bus Creator1 : BusCreator  Inputs='LVDT_H1','LVDT_H2','LVDT_H3','ACC_H1','ACC_H2','ACC_H3'
  Bus Selector : BusSelector  OutputSignals=LVDT_H1,LVDT_H2,LVDT_H3,ACC_H1,ACC_H2,ACC_H3
  COILBAL_DATE : VIS_LIB/COILBAL_DATE
  COILOUTF : Subsystem
  DAMP : Subsystem
  DAMPMODE : cdsRampMuxMatrix/Subsystem  Tag=cdsRampMuxMatrix
      settings: AttributesFormatString=%<Tag>
  DRIVEALIGN : Subsystem
  Demux{,2,6..7} (4 alike) : Demux  Outputs=3
  Demux1 : Demux  Outputs=2
  Demux9 : Demux
  EUL2COIL : cdsMuxMatrix/Subsystem  Tag=cdsMuxMatrix  Description=|
      | ADL=SUS_INMATRIX.adl
      | SCRIPT=generate_KisselButton.py 4 5 #CHANNEL# > #TARGET_DIR#/#FULL_PART_NAME#_KB.adl
      settings: AttributesFormatString=%<Tag>
  IDAMP : Subsystem
  LOCK : Subsystem
  LVDT2EUL : cdsMuxMatrix/Subsystem  Tag=cdsMuxMatrix  Description=|
      | ADL=SUS_INMATRIX.adl
      | SCRIPT=generate_KisselButton.py 4 5 #CHANNEL# > #TARGET_DIR#/#FULL_PART_NAME#_KB.adl
      settings: AttributesFormatString=%<Tag>
  LVDTINF : Subsystem
  MASTER : Subsystem
  Mux{,1,6..7} (4 alike) : Mux  Inputs=3
  Mux2 : Mux  Inputs=6
  Mux9 : Mux  Inputs=2
  SEISALIGN : cdsMuxMatrix/Subsystem  Tag=cdsMuxMatrix  Description=|
      | ADL=SUS_INMATRIX.adl
      | SCRIPT=generate_KisselButton.py 4 5 #CHANNEL# > #TARGET_DIR#/#FULL_PART_NAME#_KB.adl
      settings: AttributesFormatString=%<Tag>
  SEISFF : Subsystem
  SENSCORR : Subsystem
  SET : Subsystem
  SUMOUT : Subsystem
  Sum{,1,8..11} (6 alike) : Sum  Inputs=++|
  Sum2 : Sum  Inputs=|+-
  Sum3 : Sum  Inputs=|+-
  Sum4 : Sum  Inputs=|+-
  Sum5 : Sum  Inputs=-+|
  Sum6 : Sum  Inputs=-+|
  Sum7 : Sum  Inputs=-+|
  TEST : Subsystem
  TIDAL_L : cdsFilt/Subsystem  Tag=cdsFilt  Description=|
      | Purpose:                                                                                                                                                                                                                                  
      | Standard CDS IIR filter module.                                                                                                                                                                                                           
      |                                                                                                                                                                                                                                           
      | Operation:                                                                                                                                                                                                                                
      | Consists of 10 second order section IIR filters, plus a ramped gain stage. In FE code, also provides pre-defined test points and excitation channel inputs. The filter coefficients are defined in the LIGO system using the 'foton' tool.
      |                                                                                                                                                                                                                                           
      | Usage:                                                                                                                                                                                                                                    
      | Name the part with the desired filter module name.
      settings: AttributesFormatString=%<Tag>
  TMOLDAMP : Subsystem
  Terminator{1..3,9..10} (5 alike) : Terminator
  WATCHDOG : cdsFunctionCall/Subsystem  Tag=cdsFunctionCall  Description=inline OSEMWATCHDOG /opt/rtcds/userapps/release/vis/common/src/WATCHDOG.c
      settings: AttributesFormatString=%<Tag>\n%<Description>
  WD : Subsystem
  WDMON : TOWER_MASTER/common_blocks/WDMONMASTER
  COIL_H1_Out : Outport
  COIL_H2_Out : Outport  Port=2
  COIL_H3_Out : Outport  Port=3
  LONG_DISP_Out : Outport  Port=4
  TRANS_DISP_Out : Outport  Port=5
  YAW_DISP_Out : Outport  Port=6
  COIL_LONG_Out : Outport  Port=7
  COIL_TRANS_Out : Outport  Port=8
  COIL_YAW_Out : Outport  Port=9
  WD_BLOCK_Out : Outport  Port=10
  DAMP_STATE_Out : Outport  Port=11
  wires:
  TIDAL_L_In/1 -> TIDAL_L/1
  TIDAL_L/1 -> Sum8/1
  Sum8/1 -> Sum2/1
  GIF_ARM_L/1 -> Mux1/3
  BF_LVDT_Y_In/1 -> BFLVDAMP/3(YAW_In)
  BF_LVDT_L_In/1 -> BFLVDAMP/1(LONG_In)
  BF_LVDT_T_In/1 -> BFLVDAMP/2(TRANS_In)
  BFLVDAMP/1(LONG_Out) -> ADD/14(BFLVDAMP_L_In)
  BFLVDAMP/2(TRANS_Out) -> ADD/15(BFLVDAMP_T_In)
  BFLVDAMP/3(YAW_Out) -> ADD/16(BFLVDAMP_Y_In)
  TMOLDAMP/2(YAW_Out) -> ADD/13(TMOLDAMP_Y_In)
  TMOLDAMP/1(LONG_Out) -> ADD/12(TMOLDAMP_L_In)
  BFLVDAMP/4(DAMP_STATE_Out) -> Terminator9/1
  TM_OPLEV_Y_In/1 -> TMOLDAMP/2(YAW_In)
  TM_OPLEV_L_In/1 -> TMOLDAMP/1(LONG_In)
  TMOLDAMP/3(DAMP_STATE_Out) -> Terminator3/1
  Demux2/3 -> ADD/11(DAMP_Y_In)
  Demux2/2 -> ADD/10(DAMP_T_In)
  Demux2/1 -> ADD/9(DAMP_L_In)
  IDAMP/1(LONG_Out) -> Mux2/4
  IDAMP/2(TRANS_Out) -> Mux2/5
  IDAMP/3(YAW_Out) -> Mux2/6
  DAMP/1(LONG_Out) -> Mux2/1
  DAMP/2(TRANS_Out) -> Mux2/2
  DAMP/3(YAW_Out) -> Mux2/3
  DAMPMODE/1 -> Demux2/1
  Mux2/1 -> DAMPMODE/1
  Sum5/1 -> IDAMP/1(LONG_In)
  Sum6/1 -> IDAMP/2(TRANS_In)
  Sum7/1 -> IDAMP/3(YAW_In)
  SET/3(YAW_Out) -> Sum4/2, Sum7/1
  SET/2(TRANS_Out) -> Sum6/1, Sum3/2
  SET/1(LONG_Out) -> Sum2/2, Sum5/1
  Sum4/1 -> DAMP/3(YAW_In)
  Sum3/1 -> DAMP/2(TRANS_In)
  Sum2/1 -> DAMP/1(LONG_In)
  Demux1/1 -> SEISFF/1(LONG_In), SENSCORR/1(SEIS_L_In)
  Demux1/2 -> SEISFF/2(TRANS_In), SENSCORR/2(SEIS_T_In)
  SEISALIGN/1 -> Demux1/1
  Mux1/1 -> SEISALIGN/1
  PEM_SEIS_L_In/1 -> Mux1/1
  PEM_SEIS_T_In/1 -> Mux1/2
  ADD/3(YAW_MAIN_Out) -> SUMOUT/3(YAW_In)
  ADD/1(LONG_MAIN_Out) -> SUMOUT/1(LONG_In)
  ADD/2(TRANS_MAIN_Out) -> SUMOUT/2(TRANS_In)
  SUMOUT/2(TRANS_Out) -> Mux6/2, COIL_TRANS_Out/1
  SUMOUT/1(LONG_Out) -> Mux6/1, COIL_LONG_Out/1
  SUMOUT/3(YAW_Out) -> Mux6/3, COIL_YAW_Out/1
  [STATE_SEISFF] -> Terminator2/1
  SEISFF/1(LONG_Out) -> ADD/4(SEISFF_L_In)
  SEISFF/2(TRANS_Out) -> ADD/5(SEISFF_T_In)
  SEISFF/3(FF_STATE_Out) -> [STATE_SEISFF]
  SENSCORR/2(SC_T_Out) -> Sum1/1
  Demux/2 -> Sum1/2
  SENSCORR/1(SC_L_Out) -> Sum/1
  Demux/1 -> Sum/2
  [STATE_IDAMP] -> Terminator1/1
  IDAMP/4(DAMP_STATE_Out) -> [STATE_IDAMP]
  DAMP/4(DAMP_STATE_Out) -> [STATE_DAMP]
  BLEND/1(LONG_Out) -> Sum5/2
  LVDTINF/1(H1_Out) -> Mux/1
  LVDTINF/2(H2_Out) -> Mux/2
  LVDTINF/3(H3_Out) -> Mux/3
  Mux/1 -> LVDT2EUL/1
  LVDT2EUL/1 -> Demux/1
  Mux7/1 -> ACC2EUL/1
  ACCINF/1(H1_Out) -> Mux7/1
  ACCINF/3(H3_Out) -> Mux7/3
  ACCINF/2(H2_Out) -> Mux7/2
  ACC2EUL/1 -> Demux7/1
  Sum/1 -> BLEND/1(LVDT_L_In), LONG_DISP_Out/1, Sum8/2
  Sum1/1 -> TRANS_DISP_Out/1, BLEND/2(LVDT_T_In), Sum3/1
  Demux/3 -> YAW_DISP_Out/1, BLEND/3(LVDT_Y_In), Sum4/1
  Demux7/1 -> BLEND/4(ACC_L_In)
  Demux7/2 -> BLEND/5(ACC_T_In)
  Demux7/3 -> BLEND/6(ACC_Y_IN)
  Mux6/1 -> EUL2COIL/1
  EUL2COIL/1 -> Demux6/1
  MASTER/1(H1_Out) -> COIL_H1_Out/1
  MASTER/2(H2_Out) -> COIL_H2_Out/1
  MASTER/3(H3_Out) -> COIL_H3_Out/1
  COILOUTF/1(H1_Out) -> MASTER/1(H1_In)
  COILOUTF/2(H2_Out) -> MASTER/2(H2_In)
  COILOUTF/3(H3_Out) -> MASTER/3(H3_In)
  MASTERSW_In/1 -> MASTER/4(MASTERSWITCH)
  WD_RESET_In/1 -> Mux9/1
  WD/1(F0_AC_FLAG_Out) -> Mux9/2
  [IPSENSWD] -> Bus Selector/1
  Bus Selector/1 -> WD/1(LVDT_H1_In)  "<LVDT_H1>"
  Bus Selector/2 -> WD/2(LVDT_H2_In)  "<LVDT_H2>"
  Bus Selector/3 -> WD/3(LVDT_H3_In)  "<LVDT_H3>"
  Bus Selector/4 -> WD/4(ACC_H1_In)  "<ACC_H1>"
  Bus Selector/6 -> WD/6(ACC_H3_In)  "<ACC_H3>"
  Bus Selector/5 -> WD/5(ACC_H2_In)  "<ACC_H2>"
  Demux9/1 -> WDMON/1, [WDBLOCKFLAG]
  Demux9/2 -> WDMON/2
  Demux9/3 -> WDMON/3
  Demux9/4 -> WDMON/4
  Mux9/1 -> WATCHDOG/1
  WATCHDOG/1 -> Demux9/1
  LVDT_H1_In/1 -> Bus Creator1/1, LVDTINF/1(H1_In)
  LVDT_H2_In/1 -> Bus Creator1/2, LVDTINF/2(H2_In)
  LVDT_H3_In/1 -> Bus Creator1/3, LVDTINF/3(H3_In)
  ACC_H1_In/1 -> Bus Creator1/4, ACCINF/1(H1_In)
  ACC_H2_In/1 -> Bus Creator1/5, ACCINF/2(H2_In)
  ACC_H3_In/1 -> Bus Creator1/6, ACCINF/3(H3_In)
  Bus Creator1/1 -> [IPSENSWD]
  BLOCKFLAG/1 -> MASTER/5(BLOCKFLAG)
  BLEND/2(TRANS_Out) -> Sum6/2
  BLEND/3(YAW_Out) -> Sum7/2
  TEST/1(LONG_Out) -> ADD/6(TEST_L_In)
  TEST/2(TRANS_Out) -> ADD/7(TEST_T_In)
  TEST/3(YAW_Out) -> ADD/8(TEST_Y_In)
  COILOUTF_CTRL/1 -> COILOUTF/4(Control)
  COILOUTF_MASK/1 -> COILOUTF/5(Mask)
  [WDBLOCKFLAG] -> WD_BLOCK_Out/1
  [STATE_DAMP] -> DAMP_STATE_Out/1
  MODAL_H1_In/1 -> Sum10/1
  Demux6/1 -> Sum10/2
  Sum10/1 -> COILOUTF/1(H1_IN)
  Demux6/2 -> Sum9/2
  Sum9/1 -> COILOUTF/2(H2_IN)
  Sum11/1 -> COILOUTF/3(H3_IN)
  Demux6/3 -> Sum11/2
  MODAL_H2_In/1 -> Sum9/1
  MODAL_H3_In/1 -> Sum11/1
  ISC_L_in/1 -> LOCK/1(LONG_In)
  DRIVEALIGN/1(LONG_Out) -> ADD/1(ISC_L_In)
  LOCK/1(LONG_Out) -> DRIVEALIGN/1(LONG_In)
  LOCK/2(TRANS_Out) -> DRIVEALIGN/2(PITCH_In)
  LOCK/3(YAW_Out) -> DRIVEALIGN/3(YAW_In)
  LOCK/4(DAMP_STATE_Out) -> Terminator10/1
  ISC_T_in/1 -> LOCK/2(TRANS_In)
  ISC_Y_in/1 -> LOCK/3(YAW_In)
  DRIVEALIGN/2(PITCH_Out) -> ADD/2(ISC_T_In)
  DRIVEALIGN/3(YAW_Out) -> ADD/3(ISC_Y_In)

== system TOWER_MASTER/TOWER_MASTER/PEM ==
  SEIS_X_In : Inport
  SEIS_Y_In : Inport  Port=2
  SEIS_Z_In : Inport  Port=3
  SEISINF : Subsystem
  SEIS_X_Out : Outport
  SEIS_Y_Out : Outport  Port=2
  SEIS_Z_Out : Outport  Port=3
  wires:
  SEIS_X_In/1 -> SEISINF/1(SEIS_X_In)
  SEIS_Y_In/1 -> SEISINF/2(SEIS_Y_In)
  SEIS_Z_In/1 -> SEISINF/3(SEIS_Z_In)
  SEISINF/2(SEIS_Y_Out) -> SEIS_Y_Out/1
  SEISINF/3(SEIS_Z_Out) -> SEIS_Z_Out/1
  SEISINF/1(SEIS_X_Out) -> SEIS_X_Out/1

== system TOWER_MASTER/TOWER_MASTER/TWR_SHUTDOWN_TRIG ==
  note: AND is zero  (0) if all stages are OK
      | non-zero if BAD
  note: WDBLOCKFLAG is zero (0) if OK,
      | non-zero if BAD
  IP_WDBLOCKFLAG_In : Inport
  F0_WDBLOCKFLAG_In : Inport  Port=2
  F1_WDBLOCKFLAG_In : Inport  Port=3
  F2_WDBLOCKFLAG_In : Inport  Port=4
  F3_WDBLOCKFLAG_In : Inport  Port=5
  BF_WDBLOCKFLAG_In : Inport  Port=6
  SF_WDBLOCKFLAG_In : Inport  Port=7
  LogicalOperator1 : Logic  Operator=OR  Inputs=7  AllPortsSameDT=off  OutDataTypeStr=boolean
  STATE : cdsEpicsOut/Subsystem  Tag=cdsEpicsOutput  Description=|
      | Purpose:                                          
      | Output a FE signal to an EPICS channel.           
      |                                                   
      | Operation:                                        
      | Takes input value and passes it to EPICS record.  
      |                                                   
      | Usage:                                            
      | Name the part with the desired EPICS rrecord name.
      settings: AttributesFormatString=%<Tag>
  DACKILL_TRIG_Out : Outport
  wires:
  F2_WDBLOCKFLAG_In/1 -> LogicalOperator1/4
  F3_WDBLOCKFLAG_In/1 -> LogicalOperator1/5
  BF_WDBLOCKFLAG_In/1 -> LogicalOperator1/6
  LogicalOperator1/1 -> STATE/1
  F1_WDBLOCKFLAG_In/1 -> LogicalOperator1/3
  F0_WDBLOCKFLAG_In/1 -> LogicalOperator1/2
  IP_WDBLOCKFLAG_In/1 -> LogicalOperator1/1
  STATE/1 -> DACKILL_TRIG_Out/1
  SF_WDBLOCKFLAG_In/1 -> LogicalOperator1/7

== system TOWER_MASTER/common_blocks/BIO ==
  note: 12 Bit Word
  note: 12 Bit Word
  note: 12 Bit Word
  note: 12 Bit Word
  note: 12 Bit Word
  note: 12 Bit Word
  note: 12 Bit Word
  note: 12 Bit Word
  PI_ISC_CTRL : Inport
  PI_MON_In : Inport  Port=2
  GAS_ISC_CTRL : Inport  Port=3
  GAS_MON_In : Inport  Port=4
  BFV_ISC_CTRL : Inport  Port=5
  BFV_MON_In : Inport  Port=6
  BFH_ISC_CTRL : Inport  Port=7
  BFH_MON_In : Inport  Port=8
  BFH : STATE_BIO_MASTER/UIM_BIO_MASTER
  BFV : STATE_BIO_MASTER/UIM_BIO_MASTER
  GAS : STATE_BIO_MASTER/UIM_BIO_MASTER
  PI : STATE_BIO_MASTER/UIM_BIO_MASTER
  PI_BO_CTRL_Out : Outport
  PI_MASK_Out : Outport  Port=2
  PI_CTRL_Out : Outport  Port=3
  GAS_BO_CTRL_Out : Outport  Port=4
  GAS_MASK_Out : Outport  Port=5
  GAS_CTRL_Out : Outport  Port=6
  BFV_BO_CTRL_Out : Outport  Port=7
  BFV_MASK_Out : Outport  Port=8
  BFV_CTRL_Out : Outport  Port=9
  BFH_BO_CTRL_Out : Outport  Port=10
  BFH_MASK_Out : Outport  Port=11
  BFH_CTRL_Out : Outport  Port=12
  wires:
  BFH/3 -> BFH_BO_CTRL_Out/1
  BFH/2 -> BFH_CTRL_Out/1
  BFH/1 -> BFH_MASK_Out/1
  BFH_MON_In/1 -> BFH/2
  BFH_ISC_CTRL/1 -> BFH/1
  BFV/3 -> BFV_BO_CTRL_Out/1
  BFV/2 -> BFV_CTRL_Out/1
  BFV/1 -> BFV_MASK_Out/1
  BFV_MON_In/1 -> BFV/2
  BFV_ISC_CTRL/1 -> BFV/1
  PI/2 -> PI_CTRL_Out/1
  PI/1 -> PI_MASK_Out/1
  PI/3 -> PI_BO_CTRL_Out/1
  PI_MON_In/1 -> PI/2
  PI_ISC_CTRL/1 -> PI/1
  GAS/2 -> GAS_CTRL_Out/1
  GAS/1 -> GAS_MASK_Out/1
  GAS/3 -> GAS_BO_CTRL_Out/1
  GAS_MON_In/1 -> GAS/2
  GAS_ISC_CTRL/1 -> GAS/1

== system TOWER_MASTER/common_blocks/BIODECODE ==
  DIO_CDMON_In : Inport
  BI_MON : cdsEpicsOut/Subsystem  Tag=cdsEpicsOutput  Description=|
      | Purpose:                                          
      | Output a FE signal to an EPICS channel.           
      |                                                   
      | Operation:                                        
      | Takes input value and passes it to EPICS record.  
      |                                                   
      | Usage:                                            
      | Name the part with the desired EPICS rrecord name.
      settings: AttributesFormatString=%<Tag>
  BIO_CDMON_Out : Outport
  wires:
  DIO_CDMON_In/1 -> BI_MON/1
  BI_MON/1 -> BIO_CDMON_Out/1
